simulink model "Reglerentwurf"  (Simulink 8.7)
settings: Solver=ode45  StartTime=0.0  StopTime=10.0  RelTol=1e-3
settings Model: Creator=Oliver  LastModifiedBy=Oliver
settings DebuggingCC: UnderspecifiedInitializationDetection=Simplified  MergeDetectMultiDrivingBlocksExec=error

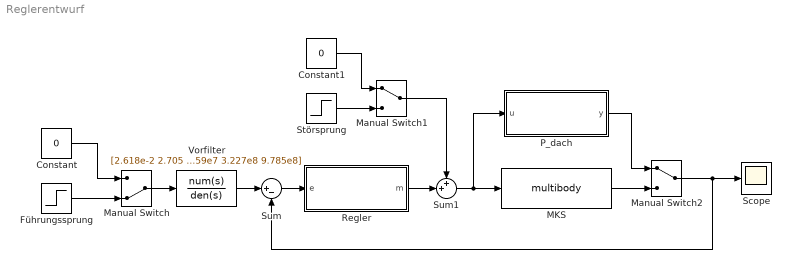
== system Reglerentwurf ==
  Constant : Constant  Value=0
  Constant1 : Constant  Value=0
  Führungssprung : Step  Time=0  SampleTime=0
  MKS : S-Function  FunctionName=multibody  Parameters='Kiethe'  SFunctionDeploymentMode=off  EnableBusSupport=off
  Manual Switch : ManualSwitch  CurrentSetting=0
  Manual Switch1 : ManualSwitch
  Manual Switch2 : ManualSwitch
  P_dach : Subsystem
  Regler : Subsystem
  Scope : Scope
  Störsprung : Step  SampleTime=0
  Sum : Sum  Inputs=|+-
  Sum1 : Sum  Inputs=++|
  Vorfilter : TransferFcn  Numerator=[2.618e-2 2.705 1.544e3 1.292e5 1.957e7 9.785e8]  Denominator=[1 3.151e2 2.132e4 7.643e5 3.559e7 3.227e8 9.785e8]
  wires:
  Vorfilter/1 -> Sum/1
  Sum/1 -> Regler/1(e)
  Manual Switch/1 -> Vorfilter/1
  Führungssprung/1 -> Manual Switch/2
  Constant/1 -> Manual Switch/1
  Sum1/1 -> P_dach/1(u), MKS/1
  Regler/1(m) -> Sum1/2
  Manual Switch1/1 -> Sum1/1
  Störsprung/1 -> Manual Switch1/2
  Constant1/1 -> Manual Switch1/1
  MKS/1 -> Manual Switch2/2
  P_dach/1(y) -> Manual Switch2/1
  Manual Switch2/1 -> Scope/1, Sum/2

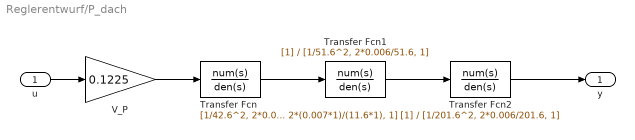
== system Reglerentwurf/P_dach ==
  u : Inport
  Transfer Fcn : TransferFcn  Numerator=[1/42.6^2, 2*0.01/42.6, 1]  Denominator=[1/(11.6*1)^2, 2*(0.007*1)/(11.6*1), 1]
  Transfer Fcn1 : TransferFcn  Denominator=[1/51.6^2, 2*0.006/51.6, 1]
  Transfer Fcn2 : TransferFcn  Denominator=[1/201.6^2, 2*0.006/201.6, 1]
  V_P : Gain  Gain=0.1225
  y : Outport
  wires:
  u/1 -> V_P/1
  V_P/1 -> Transfer Fcn/1
  Transfer Fcn/1 -> Transfer Fcn1/1
  Transfer Fcn1/1 -> Transfer Fcn2/1
  Transfer Fcn2/1 -> y/1

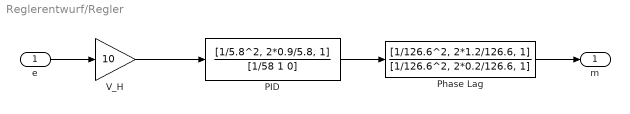
== system Reglerentwurf/Regler ==
  e : Inport
  PID : TransferFcn  Numerator=[1/5.8^2, 2*0.9/5.8, 1]  Denominator=[1/58 1 0]
  Phase Lag : TransferFcn  Numerator=[1/126.6^2, 2*1.2/126.6, 1]  Denominator=[1/126.6^2, 2*0.2/126.6, 1]
  V_H : Gain  Gain=10
  m : Outport
  wires:
  e/1 -> V_H/1
  V_H/1 -> PID/1
  Phase Lag/1 -> m/1
  PID/1 -> Phase Lag/1
